simulink model "DB_PI_1"  (R2018a)
settings: Solver=VariableStepAuto  StartTime=0.0  StopTime=10.0  RelTol=1e-3
values from neighbouring files (symbols this model uses):
  b = 1.1    [Problema1.m]    (also in Problema2.m)
  J = 15    [Problema1.m]    (also in Problema2.m)
  k = 6.8    [Problema1.m]    (also in Problema2.m = 20)
  L = 2.96e-3    (= 0.00296)    [Problema1.m]    (also in Problema2.m)
  R = 0.0435    [Problema1.m]    (also in Problema2.m)
settings Model: Creator=valen  LastModifiedBy=valen

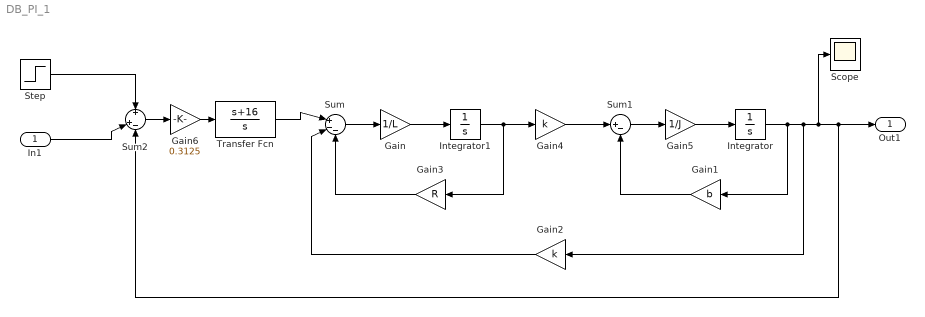
== system DB_PI_1 ==
  In1 : Inport
  Gain : Gain  Gain=1/L
  Gain1 : Gain  Gain=b
  Gain2 : Gain  Gain=k
  Gain3 : Gain  Gain=R
  Gain4 : Gain  Gain=k
  Gain5 : Gain  Gain=1/J
  Gain6 : Gain  Gain=0.3125
  Integrator : Integrator
  Integrator1 : Integrator
  Scope : Scope
  Step : Step  Time=0  Before=60  After=60  SampleTime=0
  Sum : Sum  Inputs=|+--
  Sum1 : Sum  Inputs=|+-
  Sum2 : Sum  Inputs=+|+-
  Transfer Fcn : TransferFcn  Numerator=[1 16]  Denominator=[1 0]
  Out1 : Outport
  wires:
  Sum1/1 -> Gain5/1
  Gain1/1 -> Sum1/2
  Gain3/1 -> Sum/3
  Gain2/1 -> Sum/2
  Gain5/1 -> Integrator/1
  Integrator1/1 -> Gain3/1, Gain4/1
  Gain/1 -> Integrator1/1
  Sum/1 -> Gain/1
  In1/1 -> Sum2/2
  Integrator/1 -> Gain1/1, Gain2/1, Scope/1, Sum2/3, Out1/1
  Gain4/1 -> Sum1/1
  Transfer Fcn/1 -> Sum/1
  Sum2/1 -> Gain6/1
  Gain6/1 -> Transfer Fcn/1
  Step/1 -> Sum2/1
